simulink model "SpeedModel"  (R2021b)
settings: Solver=VariableStepAuto  StartTime=0.0  StopTime=1  RelTol=1e-3
settings Model: Creator=romas  LastModifiedBy=huynh

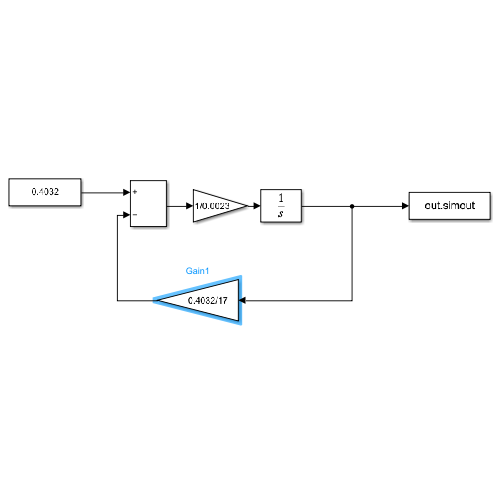
[thumbnail: Simulink's stored preview of the top-level diagram]
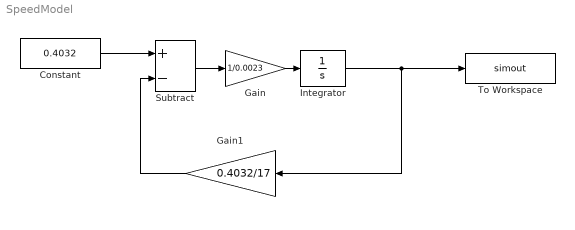
== system SpeedModel ==
  Constant : Constant  Value=0.4032
  Gain : Gain  Gain=1/0.0023
  Gain1 : Gain  Gain=0.4032/17
  Integrator : Integrator
  Subtract : Sum  Inputs=+-
  To Workspace : ToWorkspace  VariableName=simout  SaveFormat=Timeseries  SampleTime=-1
  wires:
  Constant/1 -> Subtract/1
  Gain1/1 -> Subtract/2
  Subtract/1 -> Gain/1
  Gain/1 -> Integrator/1
  Integrator/1 -> To Workspace/1, Gain1/1
